simulink library "kinematics"  (R2021b)
settings: Solver=VariableStepAuto  StartTime=0.0  StopTime=10.0  RelTol=1e-3
undefined symbols (not defined in the file or in its folder): A0, e_angles0, q0
libraries: vrlib x1
settings Model: Creator=Davide  LastModifiedBy=Davide

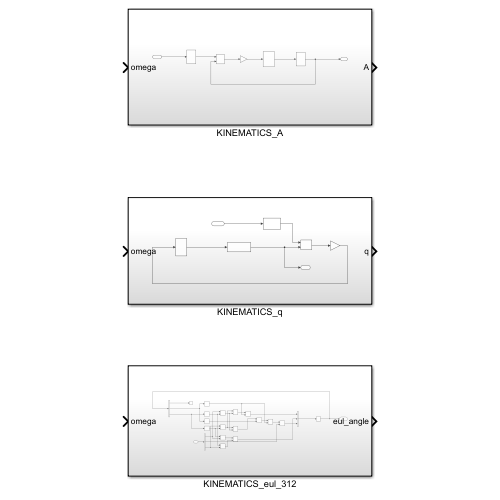
[thumbnail: Simulink's stored preview of the top-level diagram]
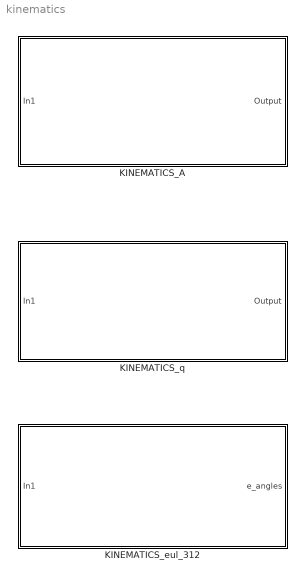
== system kinematics ==
  KINEMATICS_A : Subsystem
  KINEMATICS_eul_312 : Subsystem
  KINEMATICS_q : Subsystem

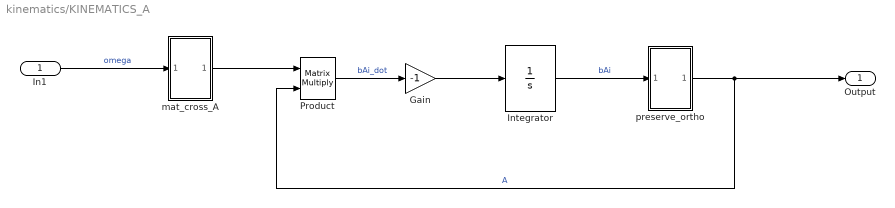
== system kinematics/KINEMATICS_A ==
  In1 : Inport
  Gain : Gain  Gain=-1
  Integrator : Integrator  InitialCondition=A0
  Product : Product  Multiplication=Matrix(*)
  mat_cross_A : Subsystem
  preserve_ortho : Subsystem
  Output : Outport
  wires:
  Integrator/1 -> preserve_ortho/1(In1)  "bAi"
  Product/1 -> Gain/1  "bAi_dot"
  In1/1 -> mat_cross_A/1(In1)  "omega"
  preserve_ortho/1(Out1) -> Output/1, Product/2  "A"
  mat_cross_A/1(Out1) -> Product/1
  Gain/1 -> Integrator/1

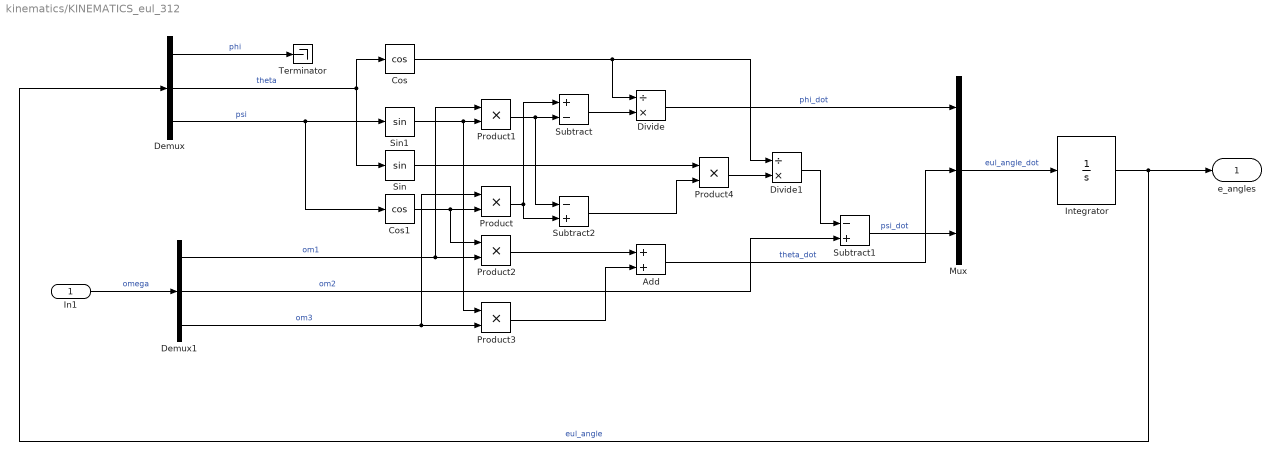
== system kinematics/KINEMATICS_eul_312 ==
  In1 : Inport
  Add : Sum
  Cos : Trigonometry  Operator=cos
  Cos1 : Trigonometry  Operator=cos
  Demux : Demux  Outputs=3
  Demux1 : Demux  Outputs=3
  Divide : Product  Inputs=/*
  Divide1 : Product  Inputs=/*
  Integrator : Integrator  InitialCondition=e_angles0
  Mux : Mux  Inputs=3
  Product{,1..4} (5 alike) : Product
  Sin : Trigonometry
  Sin1 : Trigonometry
  Subtract : Sum  Inputs=+-
  Subtract1 : Sum  Inputs=-+
  Subtract2 : Sum  Inputs=-+
  Terminator : Terminator
  e_angles : Outport
  wires:
  Add/1 -> Mux/2  "theta_dot"
  In1/1 -> Demux1/1  "omega"
  Product2/1 -> Add/1
  Cos/1 -> Divide/1, Divide1/1
  Product3/1 -> Add/2
  Divide/1 -> Mux/1  "phi_dot"
  Demux/1 -> Terminator/1  "phi"
  Integrator/1 -> Demux/1, e_angles/1  "eul_angle"
  Cos1/1 -> Product2/1, Product/2
  Sin/1 -> Product4/1
  Product1/1 -> Subtract2/1, Subtract/2
  Divide1/1 -> Subtract1/1
  Demux/3 -> Sin1/1, Cos1/1  "psi"
  Subtract/1 -> Divide/2
  Demux1/3 -> Product3/2, Product/1  "om3"
  Mux/1 -> Integrator/1  "eul_angle_dot"
  Product/1 -> Subtract2/2, Subtract/1
  Product4/1 -> Divide1/2
  Demux1/1 -> Product2/2, Product1/1  "om1"
  Demux/2 -> Cos/1, Sin/1  "theta"
  Sin1/1 -> Product3/1, Product1/2
  Subtract2/1 -> Product4/2
  Demux1/2 -> Subtract1/2  "om2"
  Subtract1/1 -> Mux/3  "psi_dot"

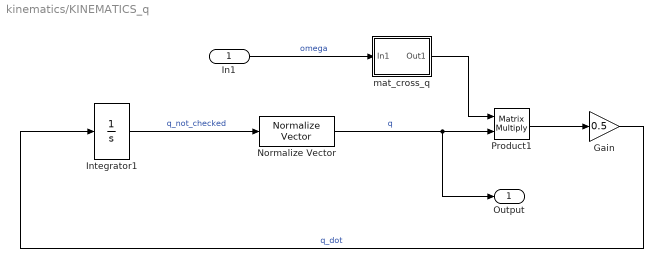
== system kinematics/KINEMATICS_q ==
  In1 : Inport
  Gain : Gain  Gain=0.5
  Integrator1 : Integrator  InitialCondition=q0
  Normalize Vector : vrlib/Utilities/Normalize Vector  maxzero=0
  Product1 : Product  Multiplication=Matrix(*)
  mat_cross_q : Subsystem
  Output : Outport
  wires:
  Gain/1 -> Integrator1/1  "q_dot"
  mat_cross_q/1(Out1) -> Product1/1
  Product1/1 -> Gain/1
  In1/1 -> mat_cross_q/1(In1)  "omega"
  Normalize Vector/1 -> Output/1, Product1/2  "q"
  Integrator1/1 -> Normalize Vector/1  "q_not_checked"

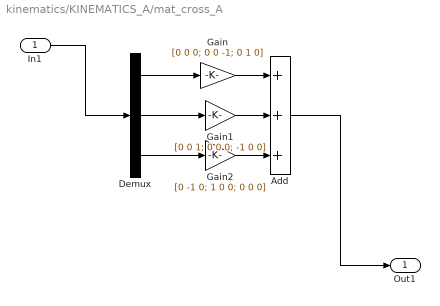
== system kinematics/KINEMATICS_A/mat_cross_A ==
  In1 : Inport
  Add : Sum  Inputs=+++
  Demux : Demux  Outputs=3
  Gain : Gain  Gain=[0 0 0; 0 0 -1; 0 1 0]
  Gain1 : Gain  Gain=[0 0 1; 0 0 0; -1 0 0]
  Gain2 : Gain  Gain=[0 -1 0; 1 0 0; 0 0 0]
  Out1 : Outport
  wires:
  In1/1 -> Demux/1
  Gain1/1 -> Add/2
  Gain2/1 -> Add/3
  Demux/2 -> Gain1/1
  Add/1 -> Out1/1
  Gain/1 -> Add/1
  Demux/3 -> Gain2/1
  Demux/1 -> Gain/1

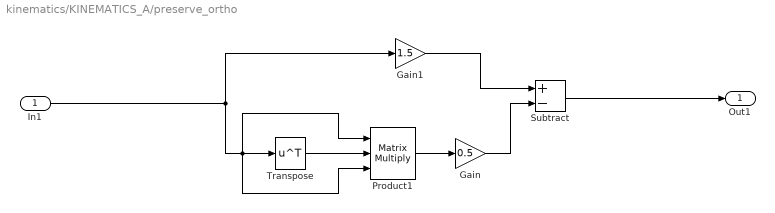
== system kinematics/KINEMATICS_A/preserve_ortho ==
  In1 : Inport
  Gain : Gain  Gain=0.5
  Gain1 : Gain  Gain=1.5
  Product1 : Product  Inputs=3  Multiplication=Matrix(*)
  Subtract : Sum  Inputs=+-
  Transpose : Math  Operator=transpose  SaturateOnIntegerOverflow=on
  Out1 : Outport
  wires:
  In1/1 -> Product1/3, Product1/1, Transpose/1, Gain1/1
  Gain1/1 -> Subtract/1
  Product1/1 -> Gain/1
  Gain/1 -> Subtract/2
  Transpose/1 -> Product1/2
  Subtract/1 -> Out1/1

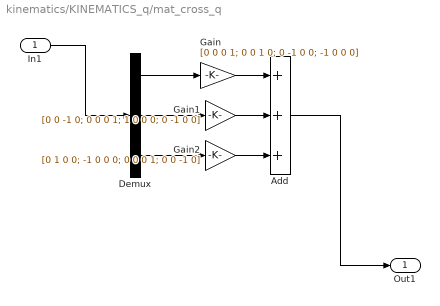
== system kinematics/KINEMATICS_q/mat_cross_q ==
  In1 : Inport
  Add : Sum  Inputs=+++
  Demux : Demux  Outputs=3
  Gain : Gain  Gain=[0 0 0 1; 0 0 1 0; 0 -1 0 0; -1 0 0 0]
  Gain1 : Gain  Gain=[0 0 -1 0; 0 0 0 1; 1 0 0 0; 0 -1 0 0]
  Gain2 : Gain  Gain=[0 1 0 0; -1 0 0 0; 0 0 0 1; 0 0 -1 0]
  Out1 : Outport
  wires:
  In1/1 -> Demux/1
  Gain1/1 -> Add/2
  Gain2/1 -> Add/3
  Demux/2 -> Gain1/1
  Add/1 -> Out1/1
  Gain/1 -> Add/1
  Demux/3 -> Gain2/1
  Demux/1 -> Gain/1
